simulink model "sl_braitenberg_light_phobic"  (R2021a)
settings: Solver=VariableStepAuto  StartTime=0.0  StopTime=200  RelTol=1e-3  EnableMultiTasking=on
undefined symbols (not defined in the file or in its folder): SE2
libraries: roblocks x1, simulink x1
settings Model: Creator=corkep  LastModifiedBy=adria
settings SolverCC: AlgebraicLoopSolver=TrustRegion
settings DataIOCC: LimitDataPoints=on  SaveFormat=Array  SaveOutput=off  SaveState=on  ReturnWorkspaceOutputs=off
settings OptimizationCC: LifeSpan=inf
settings DebuggingCC: AllowSymbolicDim=off  SFUnexpectedBacktrackingDiag=warning  SFNoUnconditionalDefaultTransitionDiag=warning  SFExecutionAtInitializationDiag=none  SFMachineParentedDataDiag=warning  ArithmeticOperatorsInVariantConditions=warning
settings HardwareCC: ProdWordSize=32
settings ModelReferenceCC: PropagateSignalLabelsOutOfModel=off
settings SFSimCC: SimUseLocalCustomCode=off  CustomCodeUndefinedFunction=UseInterfaceOnly
settings RTWCC: RTWUseLocalCustomCode=off
settings CodeAppCC: StateflowObjectComments=on
settings GRTTargetCC: TargetLangStandard=C89/C90 (ANSI)
settings ConfigComp: CovMetricSettings=dw  CovSaveCumulativeToWorkspaceVar=on  CovSaveSingleToWorkspaceVar=on  CovExternalEMLEnable=off

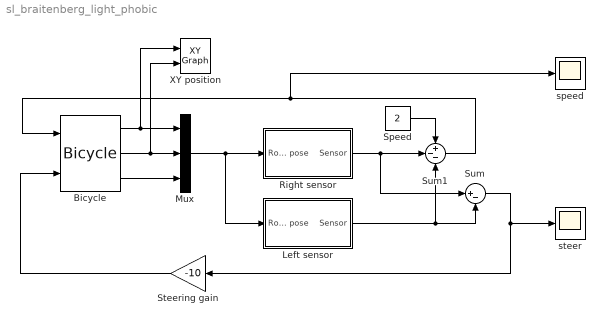
== system sl_braitenberg_light_phobic ==
  Bicycle : roblocks/Vehicles/Bicycle  vlim=1  accel=1  alim=2  steer_rate=Inf  L=1  x0=[30, 70, -pi/4]
  Left sensor : Subsystem  mask{dx=0, dy=-2, sensorfunc=@sensorfield}
      mask prompts: dx "Sensor position x"; dy "Sensor position y"; sensorfunc "Sensor function"
  Mux : Mux  Inputs=3
  Right sensor : Subsystem  mask{dx=0, dy=2, sensorfunc=@sensorfield}
      mask prompts: dx "Sensor position x"; dy "Sensor position y"; sensorfunc "Sensor function"
  Speed : Constant  Value=2
  Steering gain : Gain  Gain=-10
  Sum : Sum  Inputs=|+-
  Sum1 : Sum  Inputs=+--
  XY position : simulink/Sinks/XY Graph  xmin=0  xmax=100  ymin=0  ymax=100  st=-1
  speed : Scope
  steer : Scope
  wires:
  Bicycle/1 -> Mux/1, XY position/1
  Bicycle/2 -> Mux/2, XY position/2
  Bicycle/3 -> Mux/3
  Mux/1 -> Right sensor/1(Robot pose), Left sensor/1(Robot pose)
  Sum/1 -> steer/1, Steering gain/1
  Right sensor/1(Sensor) -> Sum/1, Sum1/2
  Left sensor/1(Sensor) -> Sum/2, Sum1/3
  Sum1/1 -> Bicycle/1, speed/1
  Speed/1 -> Sum1/1
  Steering gain/1 -> Bicycle/2

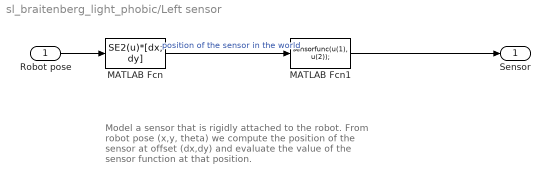
== system sl_braitenberg_light_phobic/Left sensor ==
  note: Model a sensor that is rigidly attached to the robot.
      | From robot pose (x,y, theta) we compute the position of
      | the sensor at offset (dx,dy) and evaluate the value
      | of the sensor function at that position.
  Robot pose : Inport
  MATLAB Fcn : MATLABFcn  MATLABFcn=SE2(u)*[dx; dy]
  MATLAB Fcn1 : MATLABFcn  MATLABFcn=sensorfunc(u(1), u(2));  OutputDimensions=1
  Sensor : Outport
  wires:
  Robot pose/1 -> MATLAB Fcn/1
  MATLAB Fcn/1 -> MATLAB Fcn1/1  "position of the sensor in the world"
  MATLAB Fcn1/1 -> Sensor/1

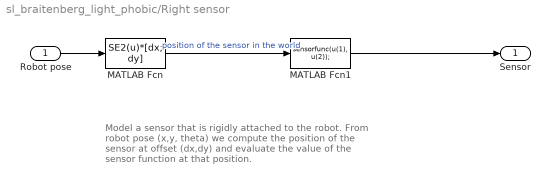
== system sl_braitenberg_light_phobic/Right sensor ==
  note: Model a sensor that is rigidly attached to the robot.
      | From robot pose (x,y, theta) we compute the position of
      | the sensor at offset (dx,dy) and evaluate the value
      | of the sensor function at that position.
  Robot pose : Inport
  MATLAB Fcn : MATLABFcn  MATLABFcn=SE2(u)*[dx; dy]
  MATLAB Fcn1 : MATLABFcn  MATLABFcn=sensorfunc(u(1), u(2));  OutputDimensions=1
  Sensor : Outport
  wires:
  Robot pose/1 -> MATLAB Fcn/1
  MATLAB Fcn/1 -> MATLAB Fcn1/1  "position of the sensor in the world"
  MATLAB Fcn1/1 -> Sensor/1
